simulink model "acrobot_zerodynamics_simulink_model"  (R2023a)
settings: Solver=ode45  StartTime=0.0  StopTime=10.0  MaxStep=1e-4  RelTol=1e-4
settings Model: Creator=MSI-  LastModifiedBy=MSI-

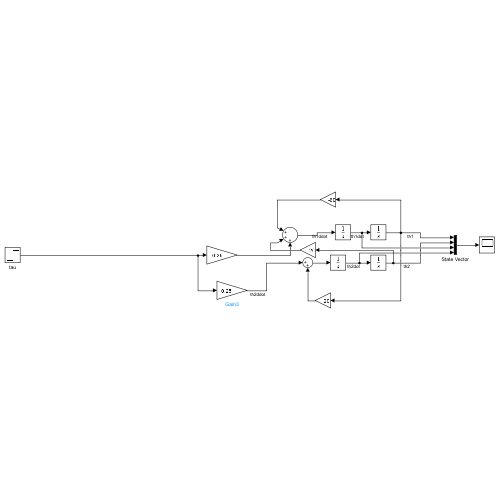
[thumbnail: Simulink's stored preview of the top-level diagram]
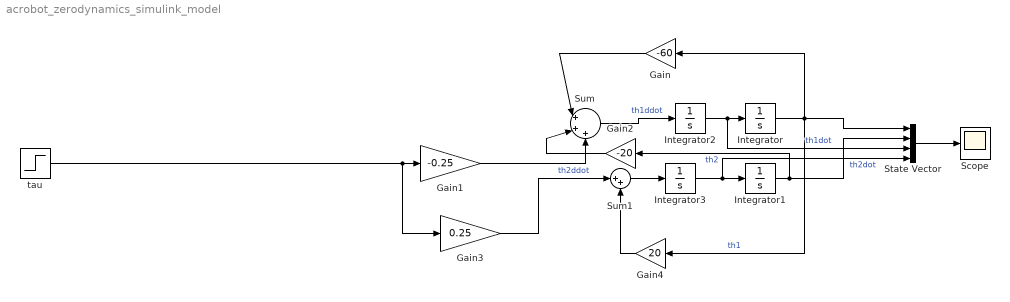
== system acrobot_zerodynamics_simulink_model ==
  Gain : Gain  Gain=-60
  Gain1 : Gain  Gain=-0.25
  Gain2 : Gain  Gain=-20
  Gain3 : Gain  Gain=0.25
  Gain4 : Gain  Gain=20
  Integrator{,1..3} (4 alike) : Integrator
  Scope : Scope
  State Vector : Mux
  Sum : Sum  Inputs=|+++
  Sum1 : Sum  Inputs=|++
  tau : Step  SampleTime=0
  wires:
  State Vector/1 -> Scope/1
  tau/1 -> Gain3/1, Gain1/1
  Integrator/1 -> Gain4/1, Gain/1, State Vector/1  "th1"
  Integrator1/1 -> Gain2/1, State Vector/2  "th2"
  Sum/1 -> Integrator2/1  "th1ddot"
  Integrator2/1 -> State Vector/3, Integrator/1  "th1dot"
  Integrator3/1 -> State Vector/4, Integrator1/1  "th2dot"
  Gain/1 -> Sum/1
  Gain1/1 -> Sum/3
  Gain2/1 -> Sum/2
  Sum1/1 -> Integrator3/1
  Gain4/1 -> Sum1/2
  Gain3/1 -> Sum1/1  "th2ddot"
